simulink model "unitVecComp_th"  (R2018b)
settings: Solver=VariableStepAuto  StartTime=0.0  StopTime=10.0  RelTol=1e-3
undefined symbols (not defined in the file): calculateRotationMatrix, params
libraries: FindUnitVectorComponents_ul x1
settings Model: Creator=asiddiq2  LastModifiedBy=asiddiq2

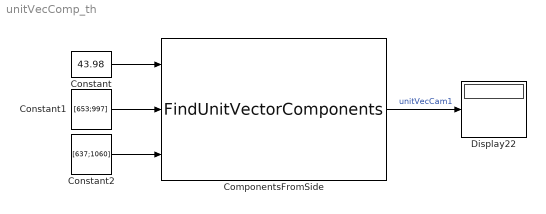
== system unitVecComp_th ==
  ComponentsFromSide : FindUnitVectorComponents_ul/FindUnitVectorComponents  cameraViewAngleVec_deg=params.cameraFOV_deg.Value  cam2GroundRotationMatrix=calculateRotationMatrix((pi/180)*params.sideCamEulAng_deg.Value(1),(pi/180)*params.sideCamEulAng_deg.Value(2),(pi/180)*params.sideCamEulAng_deg.Value(3))  imageDimensions=params.sideImageSize_px.Value
  Constant : Constant  Value=43.98
  Constant1 : Constant  Value=[653;997]  VectorParams1D=off
  Constant2 : Constant  Value=[637;1060]  VectorParams1D=off
  Display22 : Display
  wires:
  Constant/1 -> ComponentsFromSide/1
  Constant1/1 -> ComponentsFromSide/2
  Constant2/1 -> ComponentsFromSide/3
  ComponentsFromSide/1 -> Display22/1  "unitVecCam1"
